simulink model "LaunchVehicle17b"  (R2017b)
settings: Solver=VariableStepAuto  StartTime=0.0  StopTime=tSim  RelTol=1e-3
PreLoadFcn:
  | defaultModelParams;
undefined symbols (not defined in the file or in its folder): A_ol, alphaDisturbanceValue, alphaStepTime, B_ol, C_ol, den1, den2, Ki2, Kp2, num1, num2, rampDistSlope, rampInputSlope, stepTime, theta0, thetadot0, thetaPGden, thetaPGnum, thetaRGden, thetaRGnum, thetaStep, WI, windDisturbanceValue, windStepTime, Wp
libraries: simulink x2
settings Model: Creator=jyotbuch  LastModifiedBy=jyotbuch
settings OptimizationCC: LifeSpan=inf
settings DebuggingCC: SFExecutionAtInitializationDiag=none
settings CodeAppCC: StateflowObjectComments=on

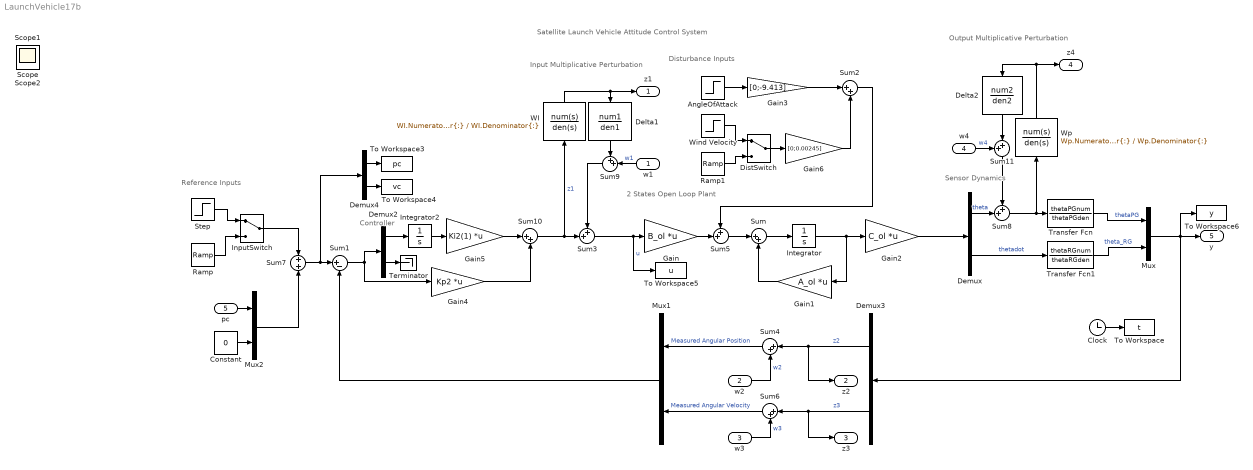
== system LaunchVehicle17b ==
  note: Input Multiplicative Perturbation
  note: Sensor Dynamics
  note: 2 States Open Loop Plant
  note: Disturbance Inputs
  note: Reference Inputs
  note: Controller
  note: Satellite Launch Vehicle Attitude Control System
  note: Output Multiplicative Perturbation
  w1 : Inport  PortDimensions=1
  w2 : Inport  Port=2  PortDimensions=1
  w3 : Inport  Port=3  PortDimensions=1
  w4 : Inport  Port=4  PortDimensions=1
  pc : Inport  Port=5  PortDimensions=1
  " WI" : TransferFcn  Numerator=WI.Numerator{:}  Denominator=WI.Denominator{:}
  " Wp" : TransferFcn  Numerator=Wp.Numerator{:}  Denominator=Wp.Denominator{:}
  AngleOfAttack : Step  Time=alphaStepTime  After=alphaDisturbanceValue  SampleTime=0
  Clock : Clock
  Constant : Constant  Value=0
  Delta1 : TransferFcn  Numerator=num1  Denominator=den1
  Delta2 : TransferFcn  Numerator=num2  Denominator=den2
  Demux{,2..4} (4 alike) : Demux  Outputs=2
  DistSwitch : ManualSwitch
  Gain : Gain  Gain=B_ol  Multiplication=Matrix(K*u)
  Gain1 : Gain  Gain=A_ol  Multiplication=Matrix(K*u)
  Gain2 : Gain  Gain=C_ol  Multiplication=Matrix(K*u)
  Gain3 : Gain  Gain=[0;-9.413]
  Gain4 : Gain  Gain=Kp2  Multiplication=Matrix(K*u) (u vector)
  Gain5 : Gain  Gain=Ki2(1)  Multiplication=Matrix(K*u) (u vector)
  Gain6 : Gain  Gain=[0;0.00245]
  InputSwitch : ManualSwitch
  Integrator : Integrator  InitialCondition=[theta0;thetadot0]
  Integrator2 : Integrator
  Mux : Mux  Inputs=2
  Mux1 : Mux  Inputs=2
  Mux2 : Mux  Inputs=2
  Ramp : simulink/Sources/Ramp  slope=rampInputSlope  start=rampInputStartTime  X0=0
  Ramp1 : simulink/Sources/Ramp  slope=rampDistSlope  start=rampDistStartTime  X0=0
  Step : Step  Time=stepTime  After=[thetaStep, 0]  SampleTime=0
  Sum{,2,4,6,10} (5 alike) : Sum  Inputs=|++
  Sum1 : Sum  Inputs=|+-
  Sum{3,5,8..9,11} (5 alike) : Sum  Inputs=++|
  Sum7 : Sum  Inputs=+|+
  Terminator : Terminator
  To Workspace : ToWorkspace  VariableName=t  SampleTime=-1
  To Workspace3 : ToWorkspace  VariableName=pc  SampleTime=-1
  To Workspace4 : ToWorkspace  VariableName=vc  SampleTime=-1
  To Workspace5 : ToWorkspace  VariableName=u  SampleTime=-1
  To Workspace6 : ToWorkspace  VariableName=y  SampleTime=-1
  Transfer Fcn : TransferFcn  Numerator=thetaPGnum  Denominator=thetaPGden
  Transfer Fcn1 : TransferFcn  Numerator=thetaRGnum  Denominator=thetaRGden
  Wind Velocity : Step  Time=windStepTime  After=windDisturbanceValue  SampleTime=0
  z1 : Outport
  z2 : Outport  Port=2
  z3 : Outport  Port=3
  z4 : Outport  Port=4
  y : Outport  Port=5
  Scope : Scope
  Scope1 : Scope
  Scope2 : Scope
  wires:
  Clock/1 -> To Workspace/1
  Integrator/1 -> Gain1/1, Gain2/1
  Gain1/1 -> Sum/2
  Sum/1 -> Integrator/1
  Sum3/1 -> To Workspace5/1, Gain/1  "u"
  Demux/2 -> Transfer Fcn1/1  "thetadot"
  Transfer Fcn/1 -> Mux/1  "thetaPG"
  Transfer Fcn1/1 -> Mux/2  "theta_RG"
  InputSwitch/1 -> Sum7/1
  w2/1 -> Sum4/2  "w2"
  w3/1 -> Sum6/2  "w3"
  Sum9/1 -> Sum3/1
  w1/1 -> Sum9/2  "w1"
  Delta1/1 -> Sum9/1
  AngleOfAttack/1 -> Gain3/1
  Ramp1/1 -> DistSwitch/2
  DistSwitch/1 -> Gain6/1
  Wind Velocity/1 -> DistSwitch/1
  Step/1 -> InputSwitch/1
  Ramp/1 -> InputSwitch/2
  Demux3/1 -> Sum4/1, z2/1  "z2"
  Demux3/2 -> z3/1, Sum6/1  "z3"
  Sum6/1 -> Mux1/2  "Measured Angular Velocity"
  Sum4/1 -> Mux1/1  "Measured Angular Position"
  pc/1 -> Mux2/1
  Sum10/1 -> Sum3/2, " WI"/1  "z1"
  Mux/1 -> To Workspace6/1, y/1, Demux3/1
  Demux2/1 -> Integrator2/1
  Integrator2/1 -> Gain5/1
  Demux2/2 -> Terminator/1
  Gain4/1 -> Sum10/2
  Sum1/1 -> Demux2/1, Gain4/1
  Sum7/1 -> Demux4/1, Sum1/1
  Mux1/1 -> Sum1/2
  Constant/1 -> Mux2/2
  Mux2/1 -> Sum7/2
  Demux4/1 -> To Workspace3/1
  Demux4/2 -> To Workspace4/1
  Gain5/1 -> Sum10/1
  Gain3/1 -> Sum2/1
  Gain6/1 -> Sum2/2
  Gain2/1 -> Demux/1
  Sum5/1 -> Sum/1
  Gain/1 -> Sum5/2
  Sum2/1 -> Sum5/1
  Demux/1 -> Sum8/2  "theta"
  Sum8/1 -> Transfer Fcn/1, " Wp"/1
  w4/1 -> Sum11/1  "w4"
  Sum11/1 -> Sum8/1
  " WI"/1 -> Delta1/1, z1/1
  " Wp"/1 -> Delta2/1, z4/1
  Delta2/1 -> Sum11/2
